simulink model "Mission_Server_Swarm_1QDrone_Unity"  (R2020b)
settings: Solver=ode2  StartTime=0.0  StopTime=inf  FixedStep=0.001  RelTol=1e-3  EnableMultiTasking=on
undefined symbols (not defined in the file): Host, qc_get_step_size
libraries: quarc_library x26, simulink x15
(part 1 of 2)
settings Model: SimulationMode=external  ExtModeTrigDuration=10000  Creator=Admin  LastModifiedBy=admin
settings SolverCC: PositivePriorityOrder=on
settings DataIOCC: ReturnWorkspaceOutputs=off
settings OptimizationCC: LifeSpan=inf
settings DebuggingCC: SFUnexpectedBacktrackingDiag=warning  SFNoUnconditionalDefaultTransitionDiag=warning  SFExecutionAtInitializationDiag=none  ArithmeticOperatorsInVariantConditions=warning
settings SFSimCC: SimUseLocalCustomCode=off  CustomCodeUndefinedFunction=UseInterfaceOnly
settings RTWCC: Description=QUARC Win64 Target  SystemTargetFile=quarc_win64.tlc  TemplateMakefile=quarc_default_tmf  RTWUseLocalCustomCode=off
settings CodeAppCC: StateflowObjectComments=on
settings STFCustomTargetCC: CPPClassGenCompliant=off
settings GRTTargetCC: TargetLangStandard=C89/C90 (ANSI)  ParMdlRefBuildCompliant=off  CompOptLevelCompliant=off  CombineOutputUpdateFcns=off  MatFileLogging=off  CPPClassGenCompliant=off  GRTInterface=on  UseToolchainInfoCompliant=off  ExtMode=on  ExtModeMexFile=quarc_comm  ExtModeMexArgs='-w -d %d -uri %u -d_IP_1 tcpip://localhost:18001'
settings ConfigComp: CovMetricSettings=dw  CovSaveCumulativeToWorkspaceVar=on  CovSaveSingleToWorkspaceVar=on  CovExternalEMLEnable=off

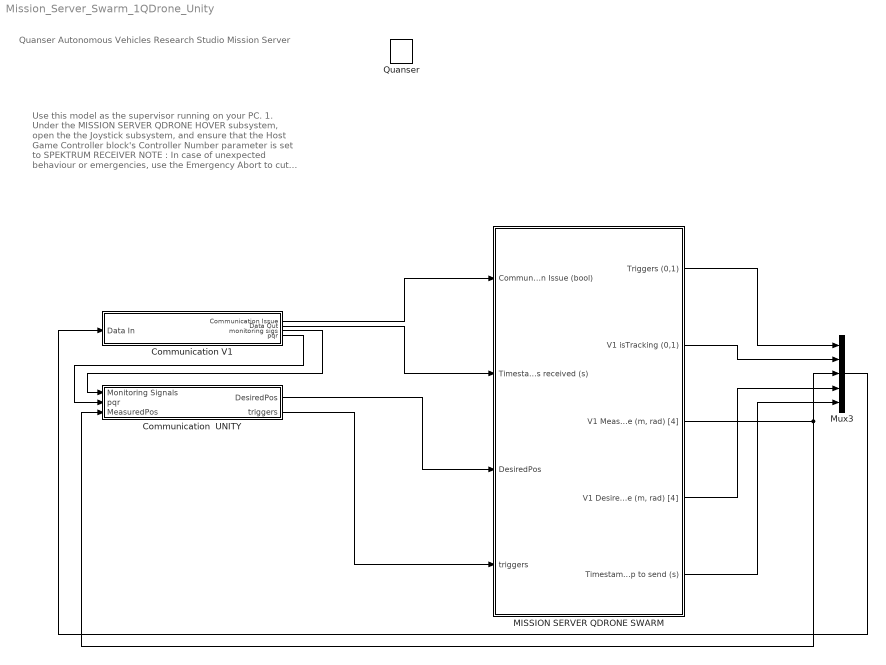
== system Mission_Server_Swarm_1QDrone_Unity ==
  note: Use this model as the supervisor running on your PC.
      |
      | 1. Under the MISSION SERVER QDRONE HOVER subsystem, open the the Joystick subsystem, and ensure that the Host Game Controller block's Controller Number parameter is set to SPEKTRUM RECEIVER
      | NOTE : In case of unexpected behaviour or emergencies, use the Emergency Abort to cut all power to the motors (this will result in the drone falling). This
      | 2. Open the Data Server (Localization) subsystem and follow the steps there.
      | 3. Under the QUARC menu, click on Build .
      | 4. Under the QUARC menu, click on Start . Wait for the model to start running.
      | 5. Ensure that the isTracking? display shows 1 and that the Joystick Issue display shows 0 (joystick must be powered ON with USB dongle attached to the PC).
      | NOTE : that the Comm Issue with Commander display SHOULD display 0 until the Commander_Stabilizer model is running. When it is running, this display should show 1.
  note: Quanser Autonomous Vehicles Research Studio
      | Mission Server
  Communication  UNITY : Subsystem
  Communication V1 : Subsystem
  MISSION SERVER QDRONE SWARM : Subsystem
  Mux3 : Mux  Inputs=5
  Quanser : quarc_library/Logos/Quanser
  wires:
  MISSION SERVER QDRONE SWARM/5(Timestamp to send (s)) -> Mux3/5
  Mux3/1 -> Communication V1/1(Data In)
  Communication V1/1(Communication Issue) -> MISSION SERVER QDRONE SWARM/1("Communication Issue (bool) ")
  Communication V1/2(Data Out) -> MISSION SERVER QDRONE SWARM/2("Timestamps received (s) ")
  MISSION SERVER QDRONE SWARM/3("V1 Measured Pose (m, rad) [4]") -> Mux3/3, Communication  UNITY/3(MeasuredPos)
  MISSION SERVER QDRONE SWARM/4("V1 Desired Pose (m, rad) [4]") -> Mux3/4
  MISSION SERVER QDRONE SWARM/1(Triggers (0,1)) -> Mux3/1
  MISSION SERVER QDRONE SWARM/2(V1 isTracking (0,1)) -> Mux3/2
  Communication V1/3(monitoring sigs) -> Communication  UNITY/1(Monitoring Signals)
  Communication  UNITY/1(DesiredPos) -> MISSION SERVER QDRONE SWARM/3(DesiredPos)
  Communication  UNITY/2(triggers) -> MISSION SERVER QDRONE SWARM/4(triggers)
  Communication V1/4(pqr) -> Communication  UNITY/2(pqr)

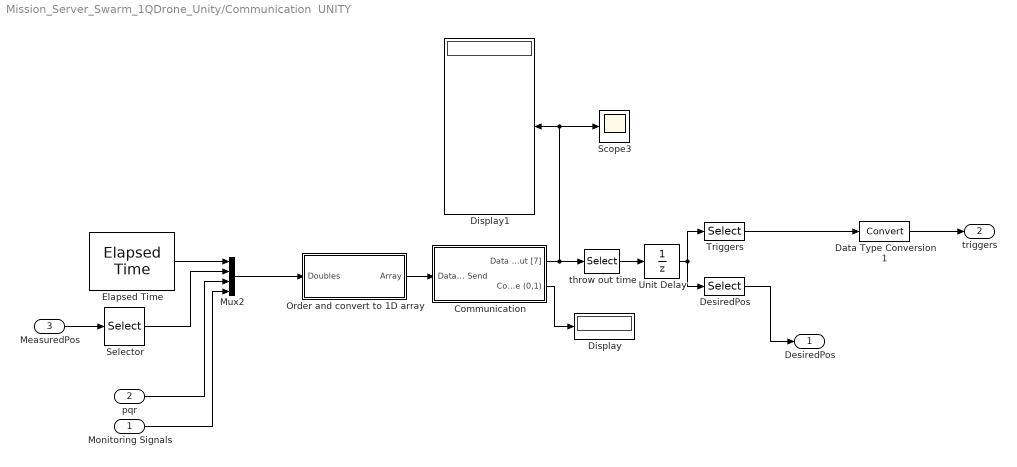
== system Mission_Server_Swarm_1QDrone_Unity/Communication  UNITY ==
  Monitoring Signals : Inport
  pqr : Inport  Port=2
  MeasuredPos : Inport  Port=3
  Communication : Subsystem
  Data Type Conversion1 : DataTypeConversion
  "DesiredPos " : Selector  InputPortWidth=7  IndexOptions=Index vector (dialog)  Indices=[4:7]  OutputSizes=1
  Display : Display
  Display1 : Display
  Elapsed Time : quarc_library/Advanced/Timing/Elapsed Time  start_src=off  sample_time=-1
      settings: SourceProductName=QUARC Targets
  Mux2 : Mux
  Order and convert to 1D array : Subsystem
  Scope3 : Scope
  Selector : Selector  InputPortWidth=4  IndexOptions=Index vector (dialog)  Indices=[1:3]  OutputSizes=1
  Triggers : Selector  InputPortWidth=7  IndexOptions=Index vector (dialog)  Indices=[1:3]  OutputSizes=1
  Unit Delay : UnitDelay  InitialCondition=zeros(1,7)  SampleTime=-1  HasFrameUpgradeWarning=on
  throw out time : Selector  InputPortWidth=8  IndexOptions=Index vector (dialog)  Indices=[2:8]  OutputSizes=1
  DesiredPos : Outport
  triggers : Outport  Port=2
  wires:
  Mux2/1 -> Order and convert to 1D array/1(Doubles)
  Elapsed Time/1 -> Mux2/1
  Order and convert to 1D array/1("Array ") -> Communication/1("Data to Send ")
  Communication/1(Data Out [7]) -> throw out time/1, Scope3/1, Display1/1
  Communication/2(Communication Issue (0,1)) -> Display/1
  MeasuredPos/1 -> Selector/1
  Monitoring Signals/1 -> Mux2/4
  "DesiredPos "/1 -> DesiredPos/1
  pqr/1 -> Mux2/3
  Triggers/1 -> Data Type Conversion1/1
  Data Type Conversion1/1 -> triggers/1
  Unit Delay/1 -> "DesiredPos "/1, Triggers/1
  throw out time/1 -> Unit Delay/1
  Selector/1 -> Mux2/2

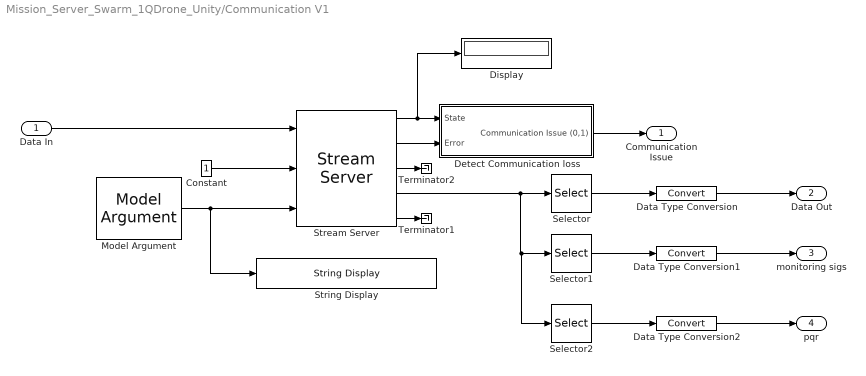
== system Mission_Server_Swarm_1QDrone_Unity/Communication V1 ==
  Data In : Inport
  Constant : Constant
  Data Type Conversion : DataTypeConversion
  Data Type Conversion1 : DataTypeConversion
  Data Type Conversion2 : DataTypeConversion
  Detect Communication loss : Subsystem
  Display : Display
  Model Argument : quarc_library/Sources/Signals/Model Argument  argument_name=d_IP_1  has_value=on  data_type_mode=Specify via dialog  data_type=char  max_length=80  variable_size=off
      settings: AttributesFormatString=(-%<argument_name>)  SourceProductName=QUARC Targets
  Selector : Selector  InputPortWidth=24  IndexOptions=Index vector (dialog)  Indices=[1]  OutputSizes=1
  Selector1 : Selector  InputPortWidth=24  IndexOptions=Index vector (dialog)  Indices=[2:21]  OutputSizes=1
  Selector2 : Selector  InputPortWidth=24  IndexOptions=Index vector (dialog)  Indices=[22:24]  OutputSizes=1
  Stream Server : quarc_library/Communications/Basic/Stream Server  uri_source=External input port  uri=tcpip://localhost:18877  apply_uri_to_all_configs=off  send_buffer_size=1460  receive_buffer_size=1460  byte_order=little endian (Intel - LSB first)  optimization=Minimum latency  send_options=Send most recent data  receive_options=Receive most recent data  default_value=zeros(1,24)  sample_time=qc_get_step_size  active=off  implementation=Use blocking I/O in a separate thread  send_fifo_size=1000  receive_fifo_size=1000  send_priority=0  receive_priority=0  send_dimensions=off  receive_dimensions=off  max_dimensions=-1  data_type=Inherited via back propagation  type_expr=BusObject
  "String Display " : quarc_library/Strings/String Display  alignment=center  display_mode=Single line  sample_time=-1  use_new=off
      settings: SourceProductName=QUARC Targets
  Terminator1 : Terminator
  Terminator2 : Terminator
  Communication Issue : Outport  VectorParamsAs1DForOutWhenUnconnected=off
  Data Out : Outport  Port=2  VectorParamsAs1DForOutWhenUnconnected=off
  monitoring sigs : Outport  Port=3
  pqr : Outport  Port=4
  wires:
  Detect Communication loss/1(Communication Issue (0,1)) -> Communication Issue/1
  Stream Server/1 -> Display/1, Detect Communication loss/1(State)
  Stream Server/2 -> Detect Communication loss/2(Error)
  Stream Server/4 -> Selector2/1, Selector1/1, Selector/1
  Model Argument/1 -> Stream Server/3, "String Display "/1
  Stream Server/5 -> Terminator1/1
  Stream Server/3 -> Terminator2/1
  Data In/1 -> Stream Server/1
  Constant/1 -> Stream Server/2
  Data Type Conversion/1 -> Data Out/1
  Selector/1 -> Data Type Conversion/1
  Data Type Conversion1/1 -> monitoring sigs/1
  Selector1/1 -> Data Type Conversion1/1
  Selector2/1 -> Data Type Conversion2/1
  Data Type Conversion2/1 -> pqr/1

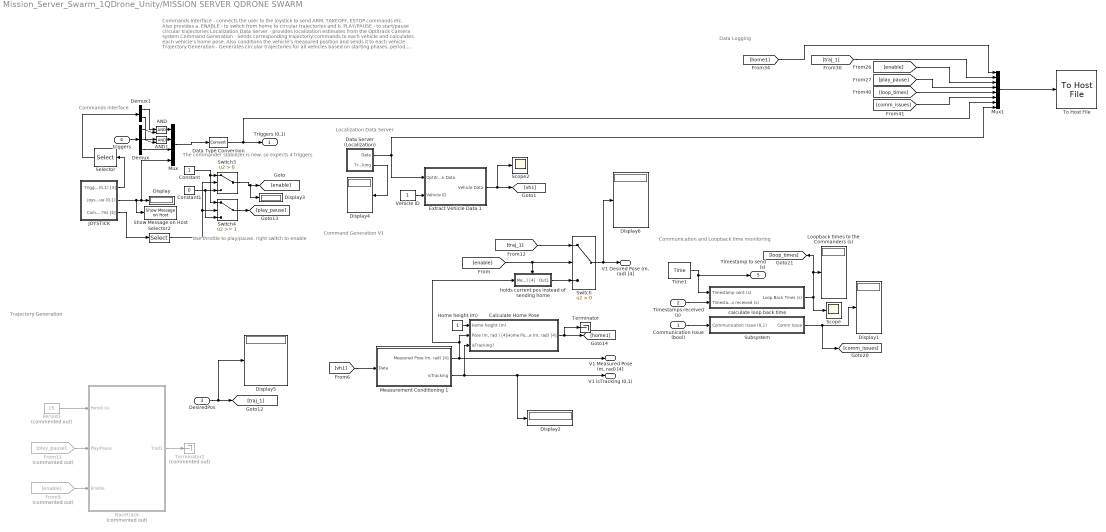
== system Mission_Server_Swarm_1QDrone_Unity/MISSION SERVER QDRONE SWARM ==
  note: The commander stabilizer is new, so expects 4 triggers
  note: Commands Interface - connects the user to the joystick to send ARM, TAKEOFF, ESTOP commands etc. Also provides a. ENABLE - to switch from home to circular trajectories and b. PLAY/PAUSE - to start/pause circular trajectories
      | Localization Data Server - provides localization estimates from the Optitrack Camera system
      | Command Generation - Sends corresponding trajectoriy commands to each vehicle and calculates each vehicle's home pose. Also conditions the vehicle's measured position and sends it to each vehicle.
      | Trajectory Generation - Generates circular trajectories for all vehicles based on starting phases, period, radus and center location. When ENABLE is low, it switches to the trajectory at the Default (m, rad) [4] input
      | Communication and Loopback time monitoring - monitors communication issues with any vehicle, and also displays the loopback time to each model (time taken to send a packet to a vehicle and receive it back immediately).
  note: Data Logging
  note: Communication and Loopback time monitoring
  note: Trajectory Generation
  note: Localization Data Server
  note: Commands Interface
  note: Command Generation V1
  note: Use throttle to play/pause, right switch to enable
  "Communication Issue (bool) " : Inport
  "Timestamps received (s) " : Inport  Port=2
  DesiredPos : Inport  Port=3
  triggers : Inport  Port=4
  AND : Logic  IconShape=distinctive  AllPortsSameDT=off  OutDataTypeStr=boolean
  AND1 : Logic  IconShape=distinctive  AllPortsSameDT=off  OutDataTypeStr=boolean
  Calculate Home Pose : Subsystem
  Constant : Constant
  Constant1 : Constant  Value=0
  "Data Server (Localization) " : Subsystem
  Data Type Conversion : DataTypeConversion
  Demux : Demux  Outputs=3
  Demux1 : Demux  Outputs=2
  Display{,1..6} (7 alike) : Display
  Extract Vehicle Data 1 : Subsystem
  From11 : From  Commented=on  GotoTag=play_pause
  From9 : From  Commented=on  GotoTag=enable
  Home height (m) : Constant
  JOYSTICK : Subsystem
  Loopback times to the Commanders (s) : Display
  Measurement Conditioning 1 : Subsystem
  Mux : Mux
  Mux1 : Mux  Inputs=8
  Period1 : Constant  Commented=on  Value=15
  Racetrack : Subsystem  Commented=on
  Scope : Scope
  Scope2 : Scope
  Selector : Selector  InputPortWidth=3  IndexOptions=Index vector (dialog)  Indices=[1:2]  OutputSizes=1
  Selector2 : Selector  InputPortWidth=4  IndexOptions=Index vector (dialog)  Indices=[1]  OutputSizes=1
  "Show Message on Host " : quarc_library/Sinks/Error Handling/Show Message on Host  message_type=Fixed error message  message_icon=Warning  message=Mission Server: Joystick Disconnected
      settings: AttributesFormatString="\"%<message>\""  SourceProductName=QUARC Targets
  Subsystem : Subsystem
  Switch : Switch  Criteria=u2 > Threshold
  Switch3 : Switch  Criteria=u2 > Threshold
  Switch4 : Switch  Threshold=1
  Terminator : Terminator
  Terminator2 : Terminator  Commented=on
  Time1 : quarc_library/Sources/Time/Time  time_source=Wall clock  sample_time=qc_get_step_size
  To Host File : quarc_library/Sinks/To Host/To Host File  file_name=saved_data/%m/%{date}_%{time}.mat  variable_name=data  decimation=1  sample_time=-1  file_format=MAT-file v.4  options=No header or footer  append=off  final_file_name=saved_data/Mission_Server_Swarm_1QDrone_Unity/18-Apr-2024_15-07-36.mat  bitrate=2000000
  Vehicle ID : Constant
  calculate loop back time : Subsystem
  holds current pos instead of sending home : Subsystem  TreatAsAtomicUnit=on
  Triggers (0,1) : Outport  VectorParamsAs1DForOutWhenUnconnected=off
  V1 isTracking (0,1) : Outport  Port=2  VectorParamsAs1DForOutWhenUnconnected=off
  "V1 Measured Pose (m, rad) [4]" : Outport  Port=3  VectorParamsAs1DForOutWhenUnconnected=off
  "V1 Desired Pose (m, rad) [4]" : Outport  Port=4  VectorParamsAs1DForOutWhenUnconnected=off
  Timestamp to send (s) : Outport  Port=5  VectorParamsAs1DForOutWhenUnconnected=off
  wires:
  "Data Server (Localization) "/2(Tracking) -> Display4/1
  "Timestamps received (s) "/1 -> calculate loop back time/2("Timestamps received (s) ")
  Vehicle ID/1 -> Extract Vehicle Data 1/2(Vehicle ID)
  Measurement Conditioning 1/2(isTracking) -> Display2/1, V1 isTracking (0,1)/1, Calculate Home Pose/3(isTracking?)
  Calculate Home Pose/1("Home Pose (m, rad) [4]") -> Terminator/1, [home1]
  Home height (m)/1 -> Calculate Home Pose/1(Home height (m))
  Switch/1 -> Display6/1, "V1 Desired Pose (m, rad) [4]"/1
  [enable] -> Switch/2, holds current pos instead of sending home/Enable
  Extract Vehicle Data 1/1(Vehicle Data) -> Scope2/1, [vh1]
  "Communication Issue (bool) "/1 -> Subsystem/1(Communication Issue (0,1))
  calculate loop back time/1("Loop Back Tmes (s) ") -> Scope/1, Loopback times to the Commanders (s)/1, [loop_times]
  Mux1/1 -> To Host File/1
  [play_pause] -> Mux1/4
  [enable] -> Mux1/3
  [traj_1] -> Mux1/2
  [home1] -> Mux1/1
  Subsystem/1(Comm Issue) -> [comm_issues], Display1/1
  [comm_issues] -> Mux1/6
  [loop_times] -> Mux1/5
  "Data Server (Localization) "/1(Data) -> Extract Vehicle Data 1/1(Optitrack Data), Mux1/8
  From9/1 -> Racetrack/3(Enable)
  Period1/1 -> Racetrack/1(Period (s))
  From11/1 -> Racetrack/2(Play/Pause)
  [vh1] -> Measurement Conditioning 1/1(Data)
  Switch4/1 -> [play_pause]
  Selector2/1 -> Switch4/2, Switch3/2
  JOYSTICK/3(Commands (%) [4]) -> Selector2/1
  JOYSTICK/2(Joystick Issue (0,1)) -> Display/1, Mux/4, "Show Message on Host "/1
  Constant1/1 -> Switch4/3, Switch3/3
  Constant/1 -> Switch3/1, Switch4/1
  Switch3/1 -> Display3/1, [enable]
  Racetrack/1(Trad1) -> Terminator2/1
  JOYSTICK/1(Triggers (0,1) [3]) -> Selector/1
  DesiredPos/1 -> Display5/1, [traj_1]
  triggers/1 -> Demux/1
  Demux/3 -> Mux/3
  Demux/1 -> AND/2
  AND/1 -> Mux/1
  Data Type Conversion/1 -> Mux1/7, Triggers (0,1)/1
  Mux/1 -> Data Type Conversion/1
  Time1/1 -> Timestamp to send (s)/1, calculate loop back time/1(Timestamp sent (s))
  holds current pos instead of sending home/1(Out1) -> Switch/3
  [traj_1] -> Switch/1
  Measurement Conditioning 1/1("Measured Pose (m, rad) [4]") -> "V1 Measured Pose (m, rad) [4]"/1, holds current pos instead of sending home/1("Measured Pose (m, rad) [4]"), Calculate Home Pose/2("Pose (m, rad ) [4]")
  Selector/1 -> Demux1/1
  Demux1/1 -> AND/1
  AND1/1 -> Mux/2
  Demux/2 -> AND1/2
  Demux1/2 -> AND1/1

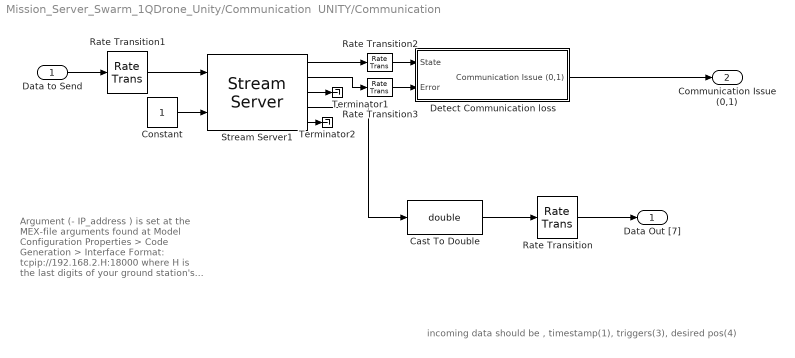
== system Mission_Server_Swarm_1QDrone_Unity/Communication  UNITY/Communication ==
  note: incoming data should be , timestamp(1), triggers(3), desired pos(4)
  note: Argument (- IP_address ) is set at the MEX-file arguments found at Model Configuration Properties > Code Generation > Interface
      |
      | Format:
      | tcpip://192.168.2.H:18000
      | where H is the last digits of your ground station's IP address (use ipconfig in a command prompt to find it out).
  "Data to Send " : Inport
  Cast To Double : DataTypeConversion  OutDataTypeStr=double
  Constant : Constant
  Detect Communication loss : Subsystem
  Rate Transition{,1..3} (4 alike) : RateTransition
  Stream Server1 : quarc_library/Communications/Basic/Stream Server  uri_source=Specify via dialog (do not evaluate)  uri=tcpip://localhost:18000?nagle='off'  apply_uri_to_all_configs=on  send_buffer_size=2048  receive_buffer_size=2048  byte_order=little endian (Intel - LSB first)  optimization=Minimum latency  send_options=Send most recent data  receive_options=Receive most recent data  default_value=zeros(1,8)  sample_time=1.0/100.0  active=on  implementation=Use blocking I/O in a separate thread  send_fifo_size=1000  receive_fifo_size=1000  send_priority=0  receive_priority=0  send_dimensions=off  receive_dimensions=off  max_dimensions=-1  data_type=single  type_expr=BusObject
      settings: AttributesFormatString="\"tcpip://localhost:18000?nagle='off'\""
  Terminator1 : Terminator
  Terminator2 : Terminator
  Data Out [7] : Outport  VectorParamsAs1DForOutWhenUnconnected=off
  Communication Issue (0,1) : Outport  Port=2  VectorParamsAs1DForOutWhenUnconnected=off
  wires:
  Stream Server1/3 -> Terminator1/1
  Detect Communication loss/1(Communication Issue (0,1)) -> Communication Issue (0,1)/1
  Cast To Double/1 -> Rate Transition/1
  Stream Server1/5 -> Terminator2/1
  Constant/1 -> Stream Server1/2
  Stream Server1/4 -> Cast To Double/1
  Rate Transition/1 -> Data Out [7]/1
  Rate Transition1/1 -> Stream Server1/1
  "Data to Send "/1 -> Rate Transition1/1
  Stream Server1/1 -> Rate Transition2/1
  Rate Transition2/1 -> Detect Communication loss/1(State)
  Stream Server1/2 -> Rate Transition3/1
  Rate Transition3/1 -> Detect Communication loss/2(Error)

== system Mission_Server_Swarm_1QDrone_Unity/Communication  UNITY/Order and convert to 1D array ==
  note: Takeoff Successful
      |
      | Flying too Low
      |
      | Flying too High
      |
      | Close to Ground
  note: Sensor Failure
  note: Command Throttle At Trim
      |
      | Command Throttle Close to 0
      |
      | Controller Throttle Close to 0
  note: Arm/Disarm
      |
      | Takeoff/Land
      |
      | Emergency Stop
      |
      | JoyStick Issue
  note: Current State
      |
      | Initializing
      |
      | Communicaiton Issue
      |
      | Tracking Issue
      |
      | Low Battery
  note: next_state
      |
      | Error
      |
      | Stop_model
  note: roll
      |
      | pitch
      |
      | yaw
  note: time
      |
      | x
      |
      | y
      |
      | z
  Doubles : Inport
  Cast To Single : DataTypeConversion  OutDataTypeStr=single
  Demux : Demux  Outputs=27
  Display : Display
  Mux : Mux  Inputs=27
  Reshape : Reshape  Commented=through
  "Array " : Outport
  wires:
  Mux/1 -> Display/1, Reshape/1
  Demux/5 -> Mux/5
  Demux/6 -> Mux/6
  Demux/7 -> Mux/7
  Demux/8 -> Mux/8
  Demux/9 -> Mux/9
  Demux/10 -> Mux/10
  Demux/11 -> Mux/11
  Demux/12 -> Mux/12
  Demux/13 -> Mux/13
  Demux/15 -> Mux/15
  Demux/16 -> Mux/16
  Demux/17 -> Mux/17
  Demux/18 -> Mux/18
  Demux/19 -> Mux/19
  Demux/20 -> Mux/20
  Demux/21 -> Mux/21
  Demux/22 -> Mux/22
  Demux/23 -> Mux/23
  Demux/24 -> Mux/24
  Demux/25 -> Mux/25
  Demux/26 -> Mux/26
  Demux/27 -> Mux/27
  Doubles/1 -> Cast To Single/1
  Demux/1 -> Mux/1
  Demux/2 -> Mux/2
  Demux/3 -> Mux/3
  Demux/4 -> Mux/4
  Demux/14 -> Mux/14
  Reshape/1 -> "Array "/1
  Cast To Single/1 -> Demux/1

== system Mission_Server_Swarm_1QDrone_Unity/Communication V1/Detect Communication loss ==
  State : Inport
  Error : Inport  Port=2
  Data Type Conversion : DataTypeConversion
  MATLAB Function : MATLAB Function  TreatAsAtomicUnit=on
  Terminator2 : Terminator
  Threshold : quarc_library/Discontinuities/Threshold  operator=>=  param_src=Specify via dialog  threshold=0.5  duration=0.1
      settings: SourceProductName=QUARC Targets
  Time : quarc_library/Sources/Time/Time  time_source=Wall clock  sample_time=qc_get_step_size
  Communication Issue (0,1) : Outport  VectorParamsAs1DForOutWhenUnconnected=off
  wires:
  Threshold/1 -> Data Type Conversion/1
  Data Type Conversion/1 -> Communication Issue (0,1)/1
  Threshold/2 -> Terminator2/1
  Time/1 -> MATLAB Function/1(time)
  State/1 -> MATLAB Function/2(state)
  MATLAB Function/1(stream_connection_loss) -> Threshold/1
  Error/1 -> MATLAB Function/3(error)

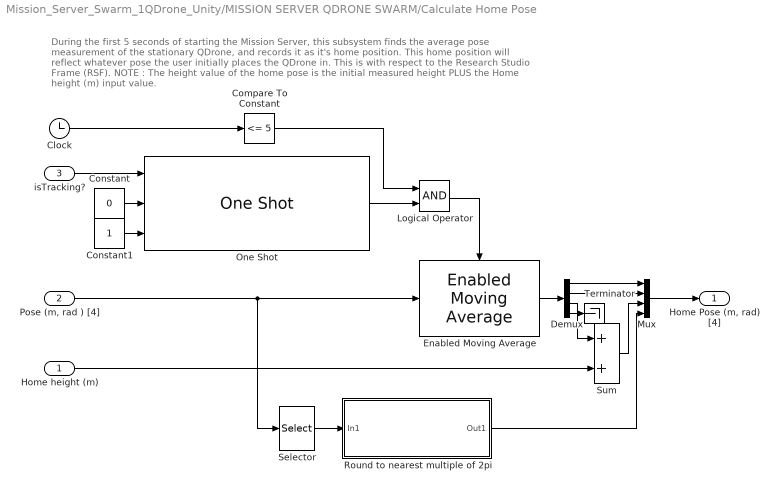
== system Mission_Server_Swarm_1QDrone_Unity/MISSION SERVER QDRONE SWARM/Calculate Home Pose ==
  note: During the first 5 seconds of starting the Mission Server, this subsystem finds the average pose measurement of the stationary QDrone,
      | and records it as it's home position. This home position will reflect whatever pose the user initially places the QDrone in.
      | This is with respect to the Research Studio Frame (RSF).
      |
      | NOTE : The height value of the home pose is the initial measured height PLUS the Home height (m) input value.
  Home height (m) : Inport
  "Pose (m, rad ) [4]" : Inport  Port=2
  isTracking? : Inport  Port=3
  Clock : Clock
  Compare To Constant : simulink/Logic and Bit Operations/Compare To Constant  relop=<=  const=5  OutDataTypeStr=boolean
  Constant : Constant  Value=0
  Constant1 : Constant
  Demux : Demux
  Enabled Moving Average : quarc_library/Discrete/Enabled Moving Average  enable_state=reset  sample_time=qc_get_step_size
      settings: SourceProductName=QUARC Targets
  Logical Operator : Logic  AllPortsSameDT=off  OutDataTypeStr=boolean
  Mux : Mux
  One Shot : quarc_library/Discontinuities/One Shot  trigger_type=Rising edge  redun_pulse=Ignore extraneous pulse  width_source=Specify via dialog  pulse_width=1/qc_get_step_size
      settings: SourceProductName=QUARC Targets
  Round to nearest multiple of 2pi : Subsystem
  Selector : Selector  InputPortWidth=4  IndexOptions=Index vector (dialog)  Indices=[4]  OutputSizes=1
  Sum : Sum
  Terminator : Terminator
  "Home Pose (m, rad) [4]" : Outport  VectorParamsAs1DForOutWhenUnconnected=off
  wires:
  Constant/1 -> One Shot/2
  Constant1/1 -> One Shot/3
  isTracking?/1 -> One Shot/1
  One Shot/1 -> Logical Operator/2
  Clock/1 -> Compare To Constant/1
  Compare To Constant/1 -> Logical Operator/1
  Logical Operator/1 -> Enabled Moving Average/Enable
  Enabled Moving Average/1 -> Demux/1
  Demux/1 -> Mux/1
  Demux/2 -> Mux/2
  Demux/3 -> Sum/1
  Sum/1 -> Mux/3
  Home height (m)/1 -> Sum/2
  Mux/1 -> "Home Pose (m, rad) [4]"/1
  Selector/1 -> Round to nearest multiple of 2pi/1(In1)
  "Pose (m, rad ) [4]"/1 -> Selector/1, Enabled Moving Average/1
  Demux/4 -> Terminator/1
  Round to nearest multiple of 2pi/1(Out1) -> Mux/4

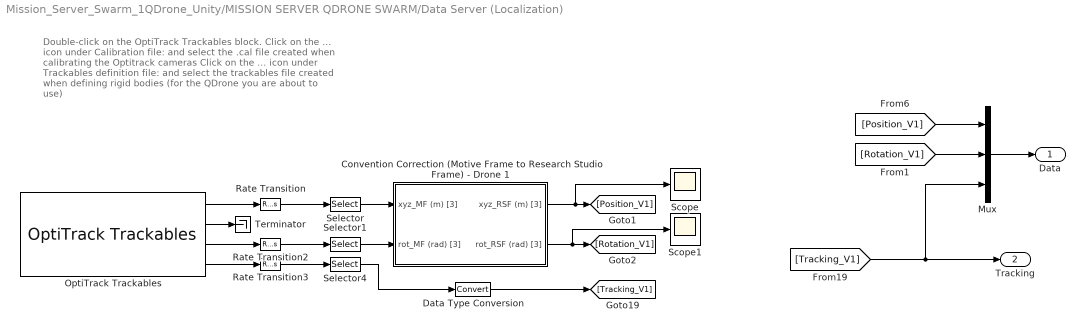
== system Mission_Server_Swarm_1QDrone_Unity/MISSION SERVER QDRONE SWARM/Data Server (Localization)  ==
  note: Double-click on the OptiTrack Trackables block.
      |
      | Click on the ... icon under Calibration file: and select the .cal file
      | created when calibrating the Optitrack cameras
      |
      | Click on the ... icon under Trackables definition file: and select
      | the trackables file created when defining rigid bodies (for the
      | QDrone you are about to use)
  Convention Correction (Motive Frame to Research Studio Frame) - Drone 1 : Subsystem
  Data Type Conversion : DataTypeConversion
  Mux : Mux  Inputs=3
  OptiTrack Trackables : quarc_library/Devices/Third-Party/NaturalPoint/OptiTrack/OptiTrack Trackables  calibration_file=C:\Users\User\Documents\OptiTrack\Session 2024-04-18\Calibration Exceptional (MeanErr 0.453 mm) 2024-04-18 2.cal  rigid_body_file=C:\Users\User\Documents\OptiTrack\Session 2020-10-01\Qdrone 043718.tra  rigid_body_ids=[1]  sample_time=qc_get_step_size*10  active=off
      settings: SourceProductName=QUARC Targets
  Rate Transition : RateTransition
  Rate Transition2 : RateTransition
  Rate Transition3 : RateTransition
  Scope : Scope
  Scope1 : Scope
  Selector : Selector  InputPortWidth=3  IndexOptions=Index vector (dialog)  Indices=[1:3]  OutputSizes=1
  Selector1 : Selector  InputPortWidth=3  IndexOptions=Index vector (dialog)  Indices=[1:3]  OutputSizes=1
  Selector4 : Selector  InputPortWidth=1  IndexOptions=Index vector (dialog)  Indices=[1]  OutputSizes=1
  Terminator : Terminator
  Data : Outport  VectorParamsAs1DForOutWhenUnconnected=off
  Tracking : Outport  Port=2  VectorParamsAs1DForOutWhenUnconnected=off
  wires:
  OptiTrack Trackables/4 -> Rate Transition3/1
  Mux/1 -> Data/1
  OptiTrack Trackables/1 -> Rate Transition/1
  OptiTrack Trackables/3 -> Rate Transition2/1
  OptiTrack Trackables/2 -> Terminator/1
  Selector/1 -> Convention Correction (Motive Frame to Research Studio Frame) - Drone 1/1(xyz_MF (m) [3])
  Selector1/1 -> Convention Correction (Motive Frame to Research Studio Frame) - Drone 1/2(rot_MF (rad) [3])
  Selector4/1 -> Data Type Conversion/1
  Rate Transition2/1 -> Selector1/1
  Rate Transition3/1 -> Selector4/1
  Rate Transition/1 -> Selector/1
  Convention Correction (Motive Frame to Research Studio Frame) - Drone 1/1(xyz_RSF (m) [3]) -> Scope/1, [Position_V1]
  [Position_V1] -> Mux/1
  Convention Correction (Motive Frame to Research Studio Frame) - Drone 1/2(rot_RSF (rad) [3]) -> Scope1/1, [Rotation_V1]
  Data Type Conversion/1 -> [Tracking_V1]
  [Tracking_V1] -> Mux/3, Tracking/1
  [Rotation_V1] -> Mux/2

== system Mission_Server_Swarm_1QDrone_Unity/MISSION SERVER QDRONE SWARM/Extract Vehicle Data 1 ==
  Optitrack Data : Inport
  Vehicle ID : Inport  Port=2
  Data Type Conversion10 : DataTypeConversion
  Data Type Conversion11 : DataTypeConversion
  Data Type Conversion9 : DataTypeConversion
  Extract Object Data : MATLAB Function  TreatAsAtomicUnit=on
  Mux1 : Mux  Inputs=3
  Reshape : Reshape
  Reshape1 : Reshape
  Reshape2 : Reshape
  Vehicle Data : Outport  VectorParamsAs1DForOutWhenUnconnected=off
  wires:
  Reshape2/1 -> Data Type Conversion9/1
  Reshape1/1 -> Data Type Conversion10/1
  Reshape/1 -> Data Type Conversion11/1
  Data Type Conversion9/1 -> Mux1/3
  Data Type Conversion10/1 -> Mux1/2
  Data Type Conversion11/1 -> Mux1/1
  Extract Object Data/2(orientation) -> Reshape1/1
  Extract Object Data/3(tracking) -> Reshape2/1
  Extract Object Data/1(position) -> Reshape/1
  Mux1/1 -> Vehicle Data/1
  Optitrack Data/1 -> Extract Object Data/1(data)
  Vehicle ID/1 -> Extract Object Data/2(index)

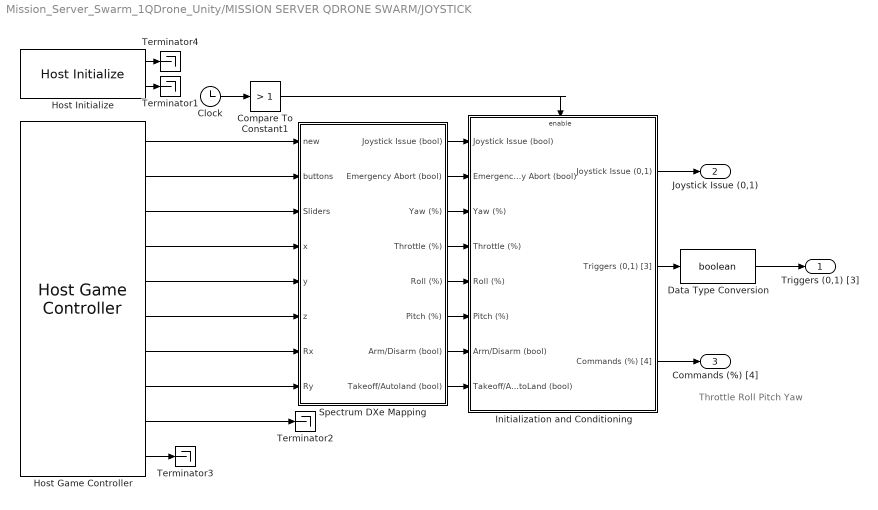
== system Mission_Server_Swarm_1QDrone_Unity/MISSION SERVER QDRONE SWARM/JOYSTICK ==
  note: Throttle
      | Roll
      | Pitch
      | Yaw
  Clock : Clock
  Compare To Constant1 : simulink/Logic and Bit Operations/Compare To Constant  relop=>  const=1  OutDataTypeStr=boolean
  Data Type Conversion : DataTypeConversion  OutDataTypeStr=boolean
  Host Game Controller : quarc_library/Devices/Peripherals/Host/Host Game Controller  object_name=Host-1  controller=1  buffer_size=20  deadzone=[]  saturation=[]  sample_time=qc_get_step_size  auto_center=off  enabled=on  debug_mode=off
      settings: SourceProductName=QUARC Targets
  Host Initialize : quarc_library/Devices/Peripherals/Host/Host Initialize  object_name=Host-1  uri_source=Use external mode communications  uri=tcpip://localhost:18001  apply_uri_to_all_configs=on  send_buffer_size=1000  receive_buffer_size=1000  thread_priority=0  run_client=on  use_window=off  window_position=[]  sample_time=qc_get_step_size  active=on
      settings: SourceProductName=QUARC Targets
  Initialization and Conditioning : Subsystem  TreatAsAtomicUnit=on
  Spectrum DXe Mapping : Subsystem
  Terminator{1..4} (4 alike) : Terminator
  Triggers (0,1) [3] : Outport  VectorParamsAs1DForOutWhenUnconnected=off
  Joystick Issue (0,1) : Outport  Port=2  VectorParamsAs1DForOutWhenUnconnected=off
  Commands (%) [4] : Outport  Port=3  VectorParamsAs1DForOutWhenUnconnected=off
  wires:
  Initialization and Conditioning/1(Joystick Issue (0,1)) -> Joystick Issue (0,1)/1
  Spectrum DXe Mapping/1(Joystick Issue (bool)) -> Initialization and Conditioning/1(Joystick Issue (bool))
  Host Game Controller/4 -> Spectrum DXe Mapping/4(x)
  Host Game Controller/5 -> Spectrum DXe Mapping/5(y)
  Host Game Controller/3 -> Spectrum DXe Mapping/3(Sliders)
  Host Game Controller/6 -> Spectrum DXe Mapping/6(z)
  Host Initialize/1 -> Terminator4/1
  Host Initialize/2 -> Terminator1/1
  Compare To Constant1/1 -> Initialization and Conditioning/Enable
  Clock/1 -> Compare To Constant1/1
  Spectrum DXe Mapping/3(Yaw (%)) -> Initialization and Conditioning/3(Yaw (%))
  Spectrum DXe Mapping/7("Arm/Disarm (bool) ") -> Initialization and Conditioning/7(Arm/Disarm (bool))
  Spectrum DXe Mapping/5(Roll (%)) -> Initialization and Conditioning/5(Roll (%))
  Spectrum DXe Mapping/4(Throttle (%)) -> Initialization and Conditioning/4(Throttle (%))
  Spectrum DXe Mapping/6(Pitch (%)) -> Initialization and Conditioning/6(Pitch (%))
  Host Game Controller/1 -> Spectrum DXe Mapping/1(new)
  Host Game Controller/2 -> Spectrum DXe Mapping/2(buttons)
  Spectrum DXe Mapping/2(Emergency Abort (bool)) -> Initialization and Conditioning/2(Emergency Abort (bool))
  Initialization and Conditioning/2(Triggers (0,1) [3]) -> Data Type Conversion/1
  Spectrum DXe Mapping/8(Takeoff/Autoland (bool)) -> Initialization and Conditioning/8(Takeoff/AutoLand (bool))
  Initialization and Conditioning/3(Commands (%) [4]) -> Commands (%) [4]/1
  Host Game Controller/7 -> Spectrum DXe Mapping/7(Rx)
  Host Game Controller/8 -> Spectrum DXe Mapping/8(Ry)
  Host Game Controller/9 -> Terminator2/1
  Host Game Controller/10 -> Terminator3/1
  Data Type Conversion/1 -> Triggers (0,1) [3]/1

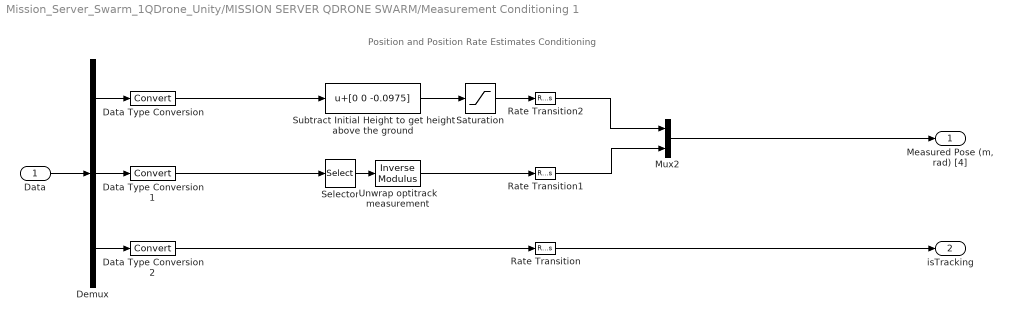
== system Mission_Server_Swarm_1QDrone_Unity/MISSION SERVER QDRONE SWARM/Measurement Conditioning 1 ==
  note: Position and Position Rate Estimates Conditioning
  Data : Inport
  Data Type Conversion : DataTypeConversion
  Data Type Conversion1 : DataTypeConversion
  Data Type Conversion2 : DataTypeConversion
  Demux : Demux  Outputs=[3 3 1]
  Mux2 : Mux  Inputs=[3 1]
  Rate Transition : RateTransition
  Rate Transition1 : RateTransition
  Rate Transition2 : RateTransition
  Saturation : Saturate  UpperLimit=[2 2 5]  LowerLimit=[-2 -2 0]
  Selector : Selector  InputPortWidth=3  IndexOptions=Index vector (dialog)  Indices=[3]  OutputSizes=1
  Subtract Initial Height to get height above the ground : Bias  Bias=[0 0 -0.0975]
  Unwrap optitrack measurement : quarc_library/Discontinuities/Inverse Modulus  modulus=2*pi  output_derivative=off  output_revolutions=off  max_x=Inf  min_x=-Inf
  "Measured Pose (m, rad) [4]" : Outport  VectorParamsAs1DForOutWhenUnconnected=off
  isTracking : Outport  Port=2  VectorParamsAs1DForOutWhenUnconnected=off
  wires:
  Demux/2 -> Data Type Conversion1/1
  Demux/1 -> Data Type Conversion/1
  Demux/3 -> Data Type Conversion2/1
  Mux2/1 -> "Measured Pose (m, rad) [4]"/1
  Data Type Conversion2/1 -> Rate Transition/1
  Data/1 -> Demux/1
  Rate Transition/1 -> isTracking/1
  Subtract Initial Height to get height above the ground/1 -> Saturation/1
  Rate Transition2/1 -> Mux2/1
  Saturation/1 -> Rate Transition2/1
  Data Type Conversion1/1 -> Selector/1
  Selector/1 -> Unwrap optitrack measurement/1
  Data Type Conversion/1 -> Subtract Initial Height to get height above the ground/1
  Unwrap optitrack measurement/1 -> Rate Transition1/1
  Rate Transition1/1 -> Mux2/2

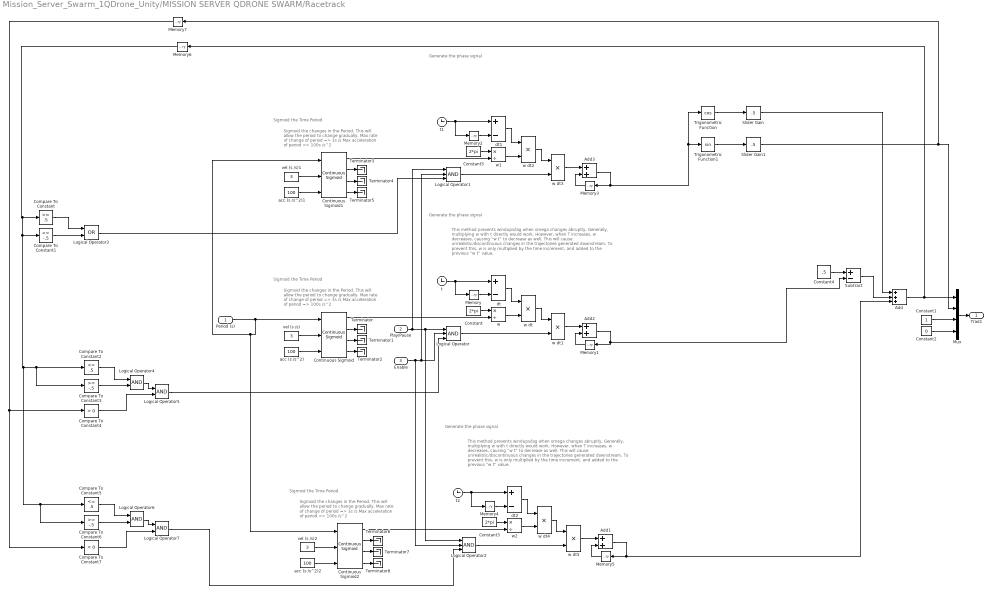
== system Mission_Server_Swarm_1QDrone_Unity/MISSION SERVER QDRONE SWARM/Racetrack ==
  note: Generate the phase signal
  note: Sigmoid the changes in the Period. This will
      | allow the period to change gradually.
      | Max rate of change of period => 3s /s
      | Max acceleration of period => 100s /s^2
  note: Sigmoid the Time Period
  note: This method prevents windups/lag when omega changes abruptly. Generally, multiplying w with t directly would work. However, when T increases, w decreases, causing "w t" to decrease as well. This will cause unrealistic/discontinuous changes in the trajectories generated downstream.
      |
      | To prevent this, w is only multiplied by the time increment, and added to the previous "w t" value.
  note: Sigmoid the changes in the Period. This will
      | allow the period to change gradually.
      | Max rate of change of period => 3s /s
      | Max acceleration of period => 100s /s^2
  note: Generate the phase signal
  note: Sigmoid the Time Period
  note: Sigmoid the changes in the Period. This will
      | allow the period to change gradually.
      | Max rate of change of period => 3s /s
      | Max acceleration of period => 100s /s^2
  note: Generate the phase signal
  note: Sigmoid the Time Period
  note: This method prevents windups/lag when omega changes abruptly. Generally, multiplying w with t directly would work. However, when T increases, w decreases, causing "w t" to decrease as well. This will cause unrealistic/discontinuous changes in the trajectories generated downstream.
      |
      | To prevent this, w is only multiplied by the time increment, and added to the previous "w t" value.
  Period (s) : Inport
  Play/Pause : Inport  Port=2
  Enable : Inport  Port=3
  Add : Sum  Inputs=+++
  Add1 : Sum
  Add2 : Sum
  Add3 : Sum
  Compare To Constant : simulink/Logic and Bit Operations/Compare To Constant  relop=>=  const=.5  OutDataTypeStr=boolean
  Compare To Constant1 : simulink/Logic and Bit Operations/Compare To Constant  relop=<=  const=-.5  OutDataTypeStr=boolean
  Compare To Constant2 : simulink/Logic and Bit Operations/Compare To Constant  relop=<=  const=.5  OutDataTypeStr=boolean
  Compare To Constant3 : simulink/Logic and Bit Operations/Compare To Constant  relop=>=  const=-.5  OutDataTypeStr=boolean
  Compare To Constant4 : simulink/Logic and Bit Operations/Compare To Constant  relop=>  const=0  OutDataTypeStr=boolean
  Compare To Constant5 : simulink/Logic and Bit Operations/Compare To Constant  relop=<=  const=.5  OutDataTypeStr=boolean
  Compare To Constant6 : simulink/Logic and Bit Operations/Compare To Constant  relop=>=  const=-.5  OutDataTypeStr=boolean
  Compare To Constant7 : simulink/Logic and Bit Operations/Compare To Constant  relop=<  const=0  OutDataTypeStr=boolean
  Constant : Constant  Value=2*pi
  Constant1 : Constant
  Constant2 : Constant  Value=0
  Constant3 : Constant  Value=2*pi
  Constant4 : Constant  Value=.5
  Constant5 : Constant  Value=2*pi
  Continuous Sigmoid : quarc_library/Sources/Sigmoids/Continuous Sigmoid  params_source=External (input ports)  max_velocity=2  max_acceleration=10  initial_position=10  initial_velocity=0  hold_off=0.5  input_sample_time=-1  output_sample_time=qc_get_step_size
      settings: SourceProductName=QUARC Targets
  Continuous Sigmoid1 : quarc_library/Sources/Sigmoids/Continuous Sigmoid  params_source=External (input ports)  max_velocity=2  max_acceleration=10  initial_position=10  initial_velocity=0  hold_off=0.5  input_sample_time=-1  output_sample_time=qc_get_step_size
      settings: SourceProductName=QUARC Targets
  Continuous Sigmoid2 : quarc_library/Sources/Sigmoids/Continuous Sigmoid  params_source=External (input ports)  max_velocity=2  max_acceleration=10  initial_position=10  initial_velocity=0  hold_off=0.5  input_sample_time=-1  output_sample_time=qc_get_step_size
      settings: SourceProductName=QUARC Targets
  Logical Operator : Logic  Inputs=3  AllPortsSameDT=off  OutDataTypeStr=boolean
  Logical Operator1 : Logic  Inputs=3  AllPortsSameDT=off  OutDataTypeStr=boolean
  Logical Operator2 : Logic  Inputs=3  AllPortsSameDT=off  OutDataTypeStr=boolean
  Logical Operator3 : Logic  Operator=OR  AllPortsSameDT=off  OutDataTypeStr=boolean
  Logical Operator{4..7} (4 alike) : Logic  AllPortsSameDT=off  OutDataTypeStr=boolean
  Memory{,1..7} (8 alike) : Memory
  Mux : Mux
  Slider Gain : simulink/Math Operations/Slider Gain  gain=.5  low=0  high=2
  Slider Gain1 : simulink/Math Operations/Slider Gain  gain=.5  low=0  high=2
  Subtract : Sum  Inputs=+-
  Terminator{,1..8} (9 alike) : Terminator
  Trigonometric Function : Trigonometry  Operator=cos
  Trigonometric Function1 : Trigonometry
  acc (s /s^2) : Constant  Value=100
  acc (s /s^2)1 : Constant  Value=100
  acc (s /s^2)2 : Constant  Value=100
  dt : Sum  Inputs=+-
  dt1 : Sum  Inputs=+-
  dt2 : Sum  Inputs=+-
  t : Clock
  t1 : Clock
  t2 : Clock
  vel (s /s) : Constant  Value=3
  vel (s /s)1 : Constant  Value=3
  vel (s /s)2 : Constant  Value=3
  w : Product  Inputs=*/
  w dt{,1..5} (6 alike) : Product
  w1 : Product  Inputs=*/
  w2 : Product  Inputs=*/
  Trad1 : Outport  VectorParamsAs1DForOutWhenUnconnected=off
  wires:
  Continuous Sigmoid/4 -> Terminator2/1
  Continuous Sigmoid/2 -> Terminator/1
  Continuous Sigmoid/3 -> Terminator1/1
  acc (s /s^2)/1 -> Continuous Sigmoid/3
  vel (s /s)/1 -> Continuous Sigmoid/2
  Memory/1 -> dt/2
  w dt/1 -> w dt1/1
  w dt1/1 -> Add2/1
  Constant/1 -> w/1
  Memory1/1 -> Add2/2
  w/1 -> w dt/2
  Continuous Sigmoid/1 -> w/2
  t/1 -> Memory/1, dt/1
  dt/1 -> w dt/1
  Play/Pause/1 -> Logical Operator1/1, Logical Operator2/1, Logical Operator/1
  Enable/1 -> Logical Operator2/2, Logical Operator1/2, Logical Operator/2
  Logical Operator/1 -> w dt1/2
  Mux/1 -> Trad1/1
  Constant2/1 -> Mux/4
  Constant1/1 -> Mux/3
  Constant4/1 -> Subtract/1
  Continuous Sigmoid1/4 -> Terminator5/1
  Add3/1 -> Trigonometric Function1/1, Trigonometric Function/1, Memory3/1
  w1/1 -> w dt2/2
  Logical Operator1/1 -> w dt3/2
  acc (s /s^2)1/1 -> Continuous Sigmoid1/3
  dt1/1 -> w dt2/1
  Continuous Sigmoid1/1 -> w1/2
  Memory2/1 -> dt1/2
  w dt3/1 -> Add3/1
  w dt2/1 -> w dt3/1
  Constant5/1 -> w1/1
  Memory3/1 -> Add3/2
  vel (s /s)1/1 -> Continuous Sigmoid1/2
  Continuous Sigmoid1/3 -> Terminator4/1
  Continuous Sigmoid1/2 -> Terminator3/1
  t1/1 -> Memory2/1, dt1/1
  Trigonometric Function/1 -> Slider Gain/1
  Trigonometric Function1/1 -> Slider Gain1/1
  Add2/1 -> Memory1/1, Subtract/2
  Subtract/1 -> Add/2
  Continuous Sigmoid2/4 -> Terminator8/1
  Add1/1 -> Add/3, Memory5/1
  w2/1 -> w dt4/2
  Logical Operator2/1 -> w dt5/2
  dt2/1 -> w dt4/1
  Continuous Sigmoid2/1 -> w2/2
  Memory4/1 -> dt2/2
  vel (s /s)2/1 -> Continuous Sigmoid2/2
  w dt5/1 -> Add1/1
  t2/1 -> Memory4/1, dt2/1
  w dt4/1 -> w dt5/1
  Constant3/1 -> w2/1
  Memory5/1 -> Add1/2
  Period (s)/1 -> Continuous Sigmoid2/1, Continuous Sigmoid1/1, Continuous Sigmoid/1
  acc (s /s^2)2/1 -> Continuous Sigmoid2/3
  Continuous Sigmoid2/3 -> Terminator7/1
  Continuous Sigmoid2/2 -> Terminator6/1
  Add/1 -> Mux/1, Memory6/1
  Slider Gain1/1 -> Memory7/1, Mux/2
  Slider Gain/1 -> Add/1
  Logical Operator3/1 -> Logical Operator1/3
  Compare To Constant/1 -> Logical Operator3/1
  Compare To Constant1/1 -> Logical Operator3/2
  Compare To Constant3/1 -> Logical Operator4/2
  Compare To Constant2/1 -> Logical Operator4/1
  Logical Operator5/1 -> Logical Operator/3
  Logical Operator4/1 -> Logical Operator5/1
  Compare To Constant4/1 -> Logical Operator5/2
  Compare To Constant6/1 -> Logical Operator6/2
  Compare To Constant5/1 -> Logical Operator6/1
  Logical Operator6/1 -> Logical Operator7/1
  Compare To Constant7/1 -> Logical Operator7/2
  Logical Operator7/1 -> Logical Operator2/3
  Memory7/1 -> Compare To Constant7/1, Compare To Constant4/1
  Memory6/1 -> Compare To Constant6/1, Compare To Constant5/1, Compare To Constant3/1, Compare To Constant2/1, Compare To Constant1/1, Compare To Constant/1

== system Mission_Server_Swarm_1QDrone_Unity/MISSION SERVER QDRONE SWARM/Subsystem ==
  note: Pass along the communication issue flag only after the connection with the vehicle model was established.
  Communication Issue (0,1) : Inport
  Logical Operator : Logic  Operator=OR  Inputs=1  AllPortsSameDT=off  OutDataTypeStr=boolean
  Product : Product
  Show Message on Host : quarc_library/Sinks/Error Handling/Show Message on Host  message_type=Fixed error message  message_icon=Warning  message=Mission Server: Communication Issue with a QDrone
      settings: AttributesFormatString="\"%<message>\""  SourceProductName=QUARC Targets
  Triggered Subsystem : Subsystem  TreatAsAtomicUnit=on
  Comm Issue : Outport  VectorParamsAs1DForOutWhenUnconnected=off
  wires:
  Communication Issue (0,1)/1 -> Product/1, Triggered Subsystem/Trigger
  Triggered Subsystem/1(Communication Issue (0,1)) -> Product/2
  Product/1 -> Comm Issue/1, Logical Operator/1
  Logical Operator/1 -> Show Message on Host/1

== system Mission_Server_Swarm_1QDrone_Unity/MISSION SERVER QDRONE SWARM/calculate loop back time ==
  Timestamp sent (s) : Inport
  "Timestamps received (s) " : Inport  Port=2
  Subtract : Sum  Inputs=+-
  "Loop Back Tmes (s) " : Outport  VectorParamsAs1DForOutWhenUnconnected=off
  wires:
  Timestamp sent (s)/1 -> Subtract/1
  "Timestamps received (s) "/1 -> Subtract/2
  Subtract/1 -> "Loop Back Tmes (s) "/1

== system Mission_Server_Swarm_1QDrone_Unity/MISSION SERVER QDRONE SWARM/holds current pos instead of sending home ==
  "Measured Pose (m, rad) [4]" : Inport
  Enable : EnablePort
  Out1 : Outport
  wires:
  "Measured Pose (m, rad) [4]"/1 -> Out1/1

== system Mission_Server_Swarm_1QDrone_Unity/Communication  UNITY/Communication/Detect Communication loss ==
  State : Inport
  Error : Inport  Port=2
  Data Type Conversion : DataTypeConversion
  MATLAB Function : MATLAB Function  TreatAsAtomicUnit=on
  Terminator2 : Terminator
  Threshold : quarc_library/Discontinuities/Threshold  operator=>=  param_src=Specify via dialog  threshold=0.5  duration=0.1
      settings: SourceProductName=QUARC Targets
  Time : quarc_library/Sources/Time/Time  time_source=Wall clock  sample_time=qc_get_step_size
  Communication Issue (0,1) : Outport  VectorParamsAs1DForOutWhenUnconnected=off
  wires:
  Threshold/1 -> Data Type Conversion/1
  Data Type Conversion/1 -> Communication Issue (0,1)/1
  Threshold/2 -> Terminator2/1
  Time/1 -> MATLAB Function/1(time)
  State/1 -> MATLAB Function/2(state)
  MATLAB Function/1(stream_connection_loss) -> Threshold/1
  Error/1 -> MATLAB Function/3(error)

== system Mission_Server_Swarm_1QDrone_Unity/MISSION SERVER QDRONE SWARM/Calculate Home Pose/Round to nearest multiple of 2pi ==
  In1 : Inport
  Abs : Abs
  Add : Sum
  Gain : Gain  Gain=2*pi
  Sign : Signum
  Subtract : Sum  Inputs=+-
  Switch : Switch  Criteria=u2 > Threshold  Threshold=pi
  fix to 2pi : Subsystem
  Out1 : Outport  VectorParamsAs1DForOutWhenUnconnected=off
  wires:
  Abs/1 -> Switch/2
  Gain/1 -> Add/2
  Switch/1 -> Out1/1
  fix to 2pi/1(Out1) -> Switch/3, Add/1, Subtract/2
  In1/1 -> fix to 2pi/1(In1), Subtract/1
  Subtract/1 -> Sign/1, Abs/1
  Sign/1 -> Gain/1
  Add/1 -> Switch/1

== system Mission_Server_Swarm_1QDrone_Unity/MISSION SERVER QDRONE SWARM/Data Server (Localization) /Convention Correction (Motive Frame to Research Studio Frame) - Drone 1 ==
  note: MF_R_RSF
  note: This subsystem converts measurements in the Motive Frame (MF)(raw optitrack) into the Research Studio Frame (RSF).
  note: RSF_R_MF
  note: XYZ in MF
  note: RPY in MF
  note: position
  note: attitude
  note: XYZ in RSF
  note: RPY in RSF
  xyz_MF (m) [3] : Inport
  rot_MF (rad) [3] : Inport  Port=2
  Inverse of Orthonormal Matrix is its Transpose : Math  Operator=transpose  SignedPower=on  SaturateOnIntegerOverflow=on
  Prevent Gimbal Lock : Subsystem
  Product : Product  Multiplication=Matrix(*)
  Product1 : Product  Multiplication=Matrix(*)
  Rotate Basis from RSF to MF : Constant  Value=[0 -1 0;0 0 1;-1 0 0]
  xyz_RSF (m) [3] : Outport  VectorParamsAs1DForOutWhenUnconnected=off
  rot_RSF (rad) [3] : Outport  Port=2  VectorParamsAs1DForOutWhenUnconnected=off
  wires:
  Rotate Basis from RSF to MF/1 -> Inverse of Orthonormal Matrix is its Transpose/1
  xyz_MF (m) [3]/1 -> Product1/2
  Inverse of Orthonormal Matrix is its Transpose/1 -> Product1/1, Product/1
  rot_MF (rad) [3]/1 -> Product/2
  Product1/1 -> xyz_RSF (m) [3]/1
  Product/1 -> Prevent Gimbal Lock/1(Attitude (rad) [3])
  Prevent Gimbal Lock/1("Attitude (rad) [3] ") -> rot_RSF (rad) [3]/1

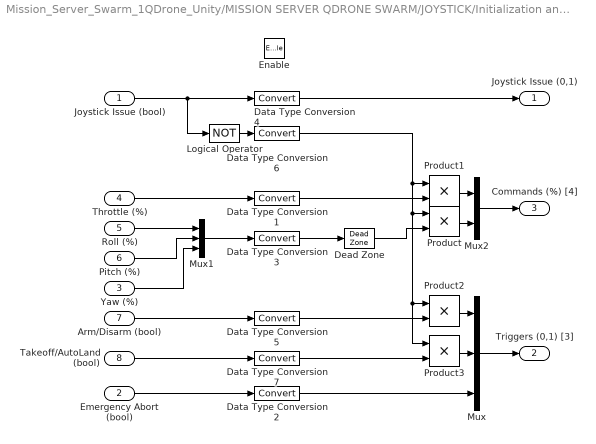
== system Mission_Server_Swarm_1QDrone_Unity/MISSION SERVER QDRONE SWARM/JOYSTICK/Initialization and Conditioning ==
  Joystick Issue (bool) : Inport
  Emergency Abort (bool) : Inport  Port=2
  Yaw (%) : Inport  Port=3
  Throttle (%) : Inport  Port=4
  Roll (%) : Inport  Port=5
  Pitch (%) : Inport  Port=6
  Arm/Disarm (bool) : Inport  Port=7
  Takeoff/AutoLand (bool) : Inport  Port=8
  Enable : EnablePort  StatesWhenEnabling=reset
  Data Type Conversion{1..7} (7 alike) : DataTypeConversion
  Dead Zone : DeadZone  LowerValue=-0.01  UpperValue=0.01  SaturateOnIntegerOverflow=on
  Logical Operator : Logic  Operator=NOT  AllPortsSameDT=off  OutDataTypeStr=boolean
  Mux : Mux  Inputs=3
  Mux1 : Mux  Inputs=3
  Mux2 : Mux  Inputs=2
  Product{,1..3} (4 alike) : Product
  Joystick Issue (0,1) : Outport  InitialOutput=0  VectorParamsAs1DForOutWhenUnconnected=off
  Triggers (0,1) [3] : Outport  Port=2  InitialOutput=0  VectorParamsAs1DForOutWhenUnconnected=off
  Commands (%) [4] : Outport  Port=3  InitialOutput=0  VectorParamsAs1DForOutWhenUnconnected=off
  wires:
  Joystick Issue (bool)/1 -> Data Type Conversion4/1, Logical Operator/1
  Mux1/1 -> Data Type Conversion3/1
  Throttle (%)/1 -> Data Type Conversion1/1
  Roll (%)/1 -> Mux1/1
  Pitch (%)/1 -> Mux1/2
  Yaw (%)/1 -> Mux1/3
  Data Type Conversion4/1 -> Joystick Issue (0,1)/1
  Emergency Abort (bool)/1 -> Data Type Conversion2/1
  Data Type Conversion3/1 -> Dead Zone/1
  Arm/Disarm (bool)/1 -> Data Type Conversion5/1
  Mux/1 -> Triggers (0,1) [3]/1
  Data Type Conversion2/1 -> Mux/3
  Logical Operator/1 -> Data Type Conversion6/1
  Product/1 -> Mux2/2
  Product1/1 -> Mux2/1
  Data Type Conversion1/1 -> Product1/2
  Dead Zone/1 -> Product/2
  Data Type Conversion6/1 -> Product1/1, Product3/1, Product2/1, Product/1
  Product2/1 -> Mux/1
  Data Type Conversion5/1 -> Product2/2
  Takeoff/AutoLand (bool)/1 -> Data Type Conversion7/1
  Product3/1 -> Mux/2
  Data Type Conversion7/1 -> Product3/2
  Mux2/1 -> Commands (%) [4]/1

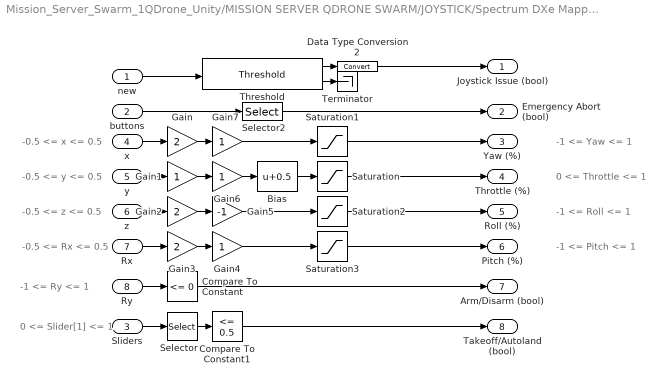
== system Mission_Server_Swarm_1QDrone_Unity/MISSION SERVER QDRONE SWARM/JOYSTICK/Spectrum DXe Mapping ==
  note: -0.5 <= x <= 0.5
  note: -1 <= Yaw <= 1
  note: -0.5 <= y <= 0.5
  note: 0 <= Throttle <= 1
  note: -0.5 <= z <= 0.5
  note: -1 <= Roll <= 1
  note: -0.5 <= Rx <= 0.5
  note: -1 <= Pitch <= 1
  note: 0 <= Slider[1] <= 1
  note: -1 <= Ry <= 1
  new : Inport
  buttons : Inport  Port=2
  Sliders : Inport  Port=3
  x : Inport  Port=4
  y : Inport  Port=5
  z : Inport  Port=6
  Rx : Inport  Port=7
  Ry : Inport  Port=8
  Bias : Bias  Bias=0.5
  Compare To Constant : simulink/Logic and Bit Operations/Compare To Constant  relop=<=  const=0  OutDataTypeStr=boolean
  Compare To Constant1 : simulink/Logic and Bit Operations/Compare To Constant  relop=<=  const=0.5  OutDataTypeStr=boolean
  Data Type Conversion2 : DataTypeConversion
  Gain : Gain  Gain=2
  Gain{1,4,6..7} (4 alike) : Gain
  Gain2 : Gain  Gain=2
  Gain3 : Gain  Gain=2
  Gain5 : Gain  Gain=-1
  Saturation : Saturate  UpperLimit=1  LowerLimit=0
  Saturation1 : Saturate  UpperLimit=1  LowerLimit=-1
  Saturation2 : Saturate  UpperLimit=1  LowerLimit=-1
  Saturation3 : Saturate  UpperLimit=1  LowerLimit=-1
  Selector : Selector  InputPortWidth=2  IndexOptions=Index vector (dialog)  Indices=[2]  OutputSizes=1
  Selector2 : Selector  InputPortWidth=32  IndexOptions=Index vector (dialog)  Indices=[1]  OutputSizes=1
  Terminator : Terminator
  Threshold : quarc_library/Discontinuities/Threshold  operator===  param_src=Specify via dialog  threshold=0  duration=1
      settings: SourceProductName=QUARC Targets
  Joystick Issue (bool) : Outport  VectorParamsAs1DForOutWhenUnconnected=off
  Emergency Abort (bool) : Outport  Port=2  VectorParamsAs1DForOutWhenUnconnected=off
  Yaw (%) : Outport  Port=3  VectorParamsAs1DForOutWhenUnconnected=off
  Throttle (%) : Outport  Port=4  VectorParamsAs1DForOutWhenUnconnected=off
  Roll (%) : Outport  Port=5  VectorParamsAs1DForOutWhenUnconnected=off
  Pitch (%) : Outport  Port=6  VectorParamsAs1DForOutWhenUnconnected=off
  "Arm/Disarm (bool) " : Outport  Port=7  VectorParamsAs1DForOutWhenUnconnected=off
  Takeoff/Autoland (bool) : Outport  Port=8  VectorParamsAs1DForOutWhenUnconnected=off
  wires:
  Compare To Constant/1 -> "Arm/Disarm (bool) "/1
  Saturation3/1 -> Pitch (%)/1
  Gain7/1 -> Saturation1/1
  Selector/1 -> Compare To Constant1/1
  Gain5/1 -> Saturation2/1
  Saturation/1 -> Throttle (%)/1
  Sliders/1 -> Selector/1
  Gain6/1 -> Bias/1
  Saturation1/1 -> Yaw (%)/1
  Gain/1 -> Gain7/1
  Gain3/1 -> Gain4/1
  Saturation2/1 -> Roll (%)/1
  Bias/1 -> Saturation/1
  Gain2/1 -> Gain5/1
  Gain1/1 -> Gain6/1
  Gain4/1 -> Saturation3/1
  z/1 -> Gain2/1
  x/1 -> Gain/1
  Ry/1 -> Compare To Constant/1
  y/1 -> Gain1/1
  Rx/1 -> Gain3/1
  Compare To Constant1/1 -> Takeoff/Autoland (bool)/1
  buttons/1 -> Selector2/1
  Threshold/2 -> Terminator/1
  Selector2/1 -> Emergency Abort (bool)/1
  Threshold/1 -> Data Type Conversion2/1
  new/1 -> Threshold/1
  Data Type Conversion2/1 -> Joystick Issue (bool)/1

== system Mission_Server_Swarm_1QDrone_Unity/MISSION SERVER QDRONE SWARM/Subsystem/Triggered Subsystem ==
  note: This looks for the first falling edge to trigger a communication issue,
      | because the mission server model starts first.
  Trigger : TriggerPort  TriggerType=falling  VariantControl=Variant
  Add : Sum
  Compare To Constant : simulink/Logic and Bit Operations/Compare To Constant  relop=>=  const=1  OutDataTypeStr=boolean
  Constant : Constant
  Memory : Memory  InheritSampleTime=on
  Communication Issue (0,1) : Outport  InitialOutput=0  VectorParamsAs1DForOutWhenUnconnected=off
  wires:
  Constant/1 -> Add/1
  Memory/1 -> Add/2
  Add/1 -> Compare To Constant/1, Memory/1
  Compare To Constant/1 -> Communication Issue (0,1)/1

== system Mission_Server_Swarm_1QDrone_Unity/MISSION SERVER QDRONE SWARM/Calculate Home Pose/Round to nearest multiple of 2pi/fix to 2pi ==
  In1 : Inport
  Constant2 : Constant  Value=2*pi
  Divide : Product  Inputs=*/
  Product : Product
  Rounding Function : Rounding  Operator=fix
  Out1 : Outport  VectorParamsAs1DForOutWhenUnconnected=off
  wires:
  Constant2/1 -> Product/2, Divide/2
  Rounding Function/1 -> Product/1
  Product/1 -> Out1/1
  Divide/1 -> Rounding Function/1
  In1/1 -> Divide/1
